simulink subsystem "Mk3Serial"  (R2024a)
settings: Solver=VariableStepAuto  StartTime=0.0  StopTime=10.0  RelTol=1e-3
undefined symbols (not defined in the file): MCU_Ts
libraries: simulink x1
settings Model: DataDictionary=neck_mk3.sldd  EnableAccessToBaseWorkspace=off  Creator=upattacini  LastModifiedBy=upattacini

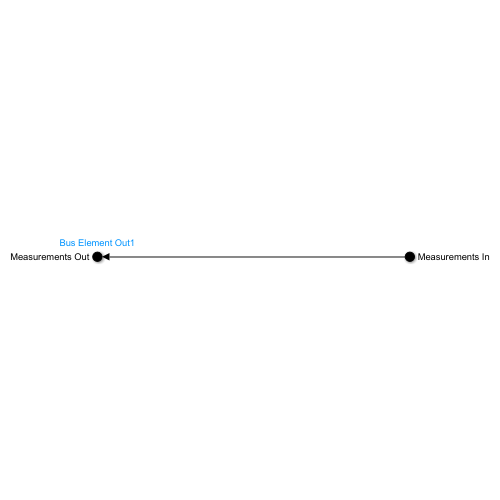
[thumbnail: Simulink's stored preview of the top-level diagram]
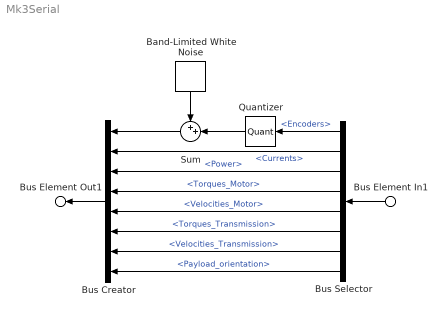
== system Mk3Serial ==
  Bus Element In1 : Inport  PortName=Measurements In
  Band-Limited White Noise : simulink/Sources/Band-Limited White Noise  Cov=(360/2^12 * 0.5)^2 * MCU_Ts  Ts=MCU_Ts  seed=[23341]
  Bus Creator : BusCreator  Inputs=8  OutDataTypeStr=Bus: Data_Measurements  NonVirtualBus=on
      settings: InheritFromInputs=off
  Bus Selector : BusSelector  OutputSignals=Encoders,Currents,Power,Torques_Motor,Velocities_Motor,Torques_Transmission,Velocities_Transmission,Payload_orientation
  Quantizer : Quantizer  QuantizationInterval=360/2^14
  Sum : Sum  Inputs=++|
  Bus Element Out1 : Outport  PortName=Measurements Out
  wires:
  Bus Element In1/1 -> Bus Selector/1
  Bus Creator/1 -> Bus Element Out1/1
  Bus Selector/1 -> Quantizer/1  "<Encoders>"
  Bus Selector/2 -> Bus Creator/2  "<Currents>"
  Bus Selector/3 -> Bus Creator/3  "<Power>"
  Bus Selector/4 -> Bus Creator/4  "<Torques_Motor>"
  Bus Selector/5 -> Bus Creator/5  "<Velocities_Motor>"
  Bus Selector/6 -> Bus Creator/6  "<Torques_Transmission>"
  Bus Selector/7 -> Bus Creator/7  "<Velocities_Transmission>"
  Bus Selector/8 -> Bus Creator/8  "<Payload_orientation>"
  Quantizer/1 -> Sum/2
  Sum/1 -> Bus Creator/1
  Band-Limited White Noise/1 -> Sum/1
